simulink model "DC_motor_PID"  (R2024a)
settings: Solver=VariableStepAuto  StartTime=0.0  StopTime=10.0  RelTol=1e-3
libraries: simulink_extras x4, nesl_utility x4, fl_lib x2
settings Model: Creator=fuad  LastModifiedBy=fuad

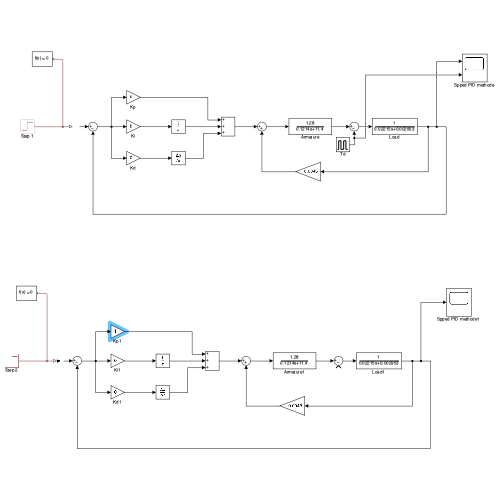
[thumbnail: Simulink's stored preview of the top-level diagram]
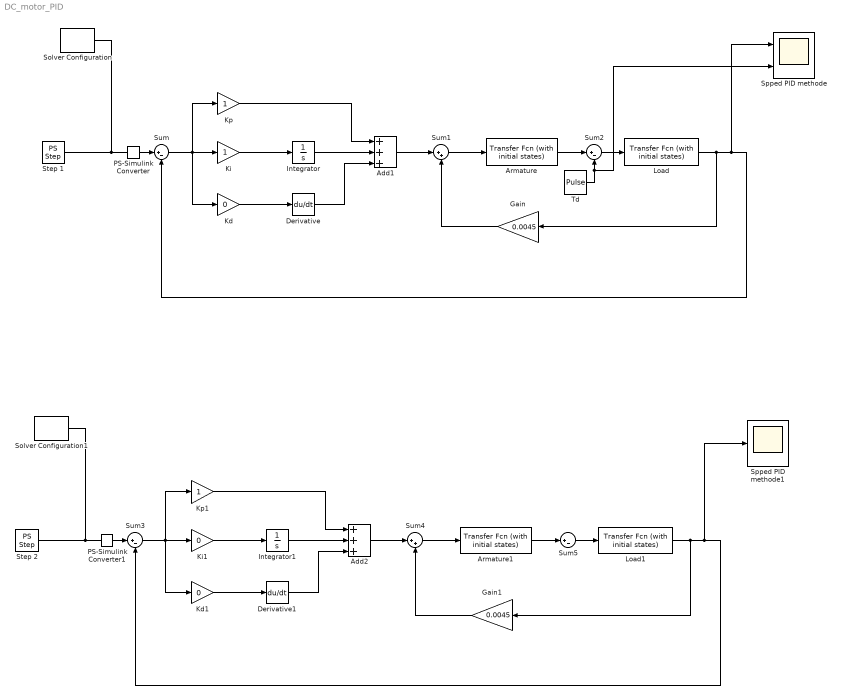
== system DC_motor_PID ==
  Add1 : Sum  Inputs=+++
  Add2 : Sum  Inputs=+++
  Armature : simulink_extras/Additional Linear/Transfer Fcn (with initial states)  N=[1.28]  D="[0.1214  11.4]"  X0=.0
  Armature1 : simulink_extras/Additional Linear/Transfer Fcn (with initial states)  N=[1.28]  D="[0.1214  11.4]"  X0=.0
  Derivative : Derivative
  Derivative1 : Derivative
  Gain : Gain  Gain=0.0045
  Gain1 : Gain  Gain=0.0045
  Integrator : Integrator
  Integrator1 : Integrator
  Kd : Gain  Gain=0
  Kd1 : Gain  Gain=0
  Ki : Gain
  Ki1 : Gain  Gain=0
  Kp : Gain
  Kp1 : Gain
  Load : simulink_extras/Additional Linear/Transfer Fcn (with initial states)  N=[1]  D="[0.02215  0.002953]"  X0=.0
  Load1 : simulink_extras/Additional Linear/Transfer Fcn (with initial states)  N=[1]  D="[0.02215  0.002953]"  X0=.0
  PS-Simulink Converter : nesl_utility/PS-Simulink Converter  PhysicalDomain=network_engine_domain  SubClassName=ps_output  LeftPortType=input  RightPortType=output  PseudoPeriodic=off  Frequencies=[]  VectorFormat=inherit  Unit=inherit  AffineConversion=off
  PS-Simulink Converter1 : nesl_utility/PS-Simulink Converter  PhysicalDomain=network_engine_domain  SubClassName=ps_output  LeftPortType=input  RightPortType=output  PseudoPeriodic=off  Frequencies=[]  VectorFormat=inherit  Unit=inherit  AffineConversion=off
  Solver Configuration : nesl_utility/Solver Configuration  PhysicalDomain=network_engine_domain  SubClassName=solver  LeftPortType=input  RightPortType=generic  Tones=[]  Harmonics=[]  SimulateNoise=off  Profile=off  UseLocalSampling=off  EnableSwitchedLinearOptims=on  FrequencyDomain=off  UseCCode=off  RelTol=0.001  AbsTol=0.001  MinStep=1e-09  ToWorkspace=off  RevertToSquareIcSolve=off  NumHomotopyIterations=100  PhasorMode=off  PhasorModeNumHarmonics=1  ConsistencySolver=NEWTON_XTOL_AFTER_FTOL  IndexReductionMethod=DerivativeReplacement  DoDC=off  ResidualTolerance=1e-09  ConsistencyTolSource=GLOBAL  ConsistencyAbsTol=0.001  ConsistencyRelTol=0.001  ConsistencyTolFactor=0.001  UseLocalSolver=off  LocalSolverChoice=NE_BACKWARD_EULER_ADVANCER  ResolveIndetEquations=on  FunctionEvalNumThread=1  LocalSolverSampleTime=0.001  DoFixedCost=off  MaxNonlinIter=3  MaxModeIter=2  ComputeImpulses=off  ImpulseIterations=2  LinearAlgebra=auto  LinearAlgebraNumThread=0  EquationFormulation=NE_TIME_EF  DelaysMemoryBudget=1024  AutomaticFiltering=on  FilteringTimeConstant=0.001  PartitionStorageMethod=AS_NEEDED  PartitionMemoryBudget=1024  PartitionMethod=ROBUST  MultibodyUseLocalSolver=off  MultibodyLocalSolverChoice=ODE1  MultibodyLocalSolverSampleTime=0.001
  Solver Configuration1 : nesl_utility/Solver Configuration  PhysicalDomain=network_engine_domain  SubClassName=solver  LeftPortType=input  RightPortType=generic  Tones=[]  Harmonics=[]  SimulateNoise=off  Profile=off  UseLocalSampling=off  EnableSwitchedLinearOptims=on  FrequencyDomain=off  UseCCode=off  RelTol=0.001  AbsTol=0.001  MinStep=1e-09  ToWorkspace=off  RevertToSquareIcSolve=off  NumHomotopyIterations=100  PhasorMode=off  PhasorModeNumHarmonics=1  ConsistencySolver=NEWTON_XTOL_AFTER_FTOL  IndexReductionMethod=DerivativeReplacement  DoDC=off  ResidualTolerance=1e-09  ConsistencyTolSource=GLOBAL  ConsistencyAbsTol=0.001  ConsistencyRelTol=0.001  ConsistencyTolFactor=0.001  UseLocalSolver=off  LocalSolverChoice=NE_BACKWARD_EULER_ADVANCER  ResolveIndetEquations=on  FunctionEvalNumThread=1  LocalSolverSampleTime=0.001  DoFixedCost=off  MaxNonlinIter=3  MaxModeIter=2  ComputeImpulses=off  ImpulseIterations=2  LinearAlgebra=auto  LinearAlgebraNumThread=0  EquationFormulation=NE_TIME_EF  DelaysMemoryBudget=1024  AutomaticFiltering=on  FilteringTimeConstant=0.001  PartitionStorageMethod=AS_NEEDED  PartitionMemoryBudget=1024  PartitionMethod=ROBUST  MultibodyUseLocalSolver=off  MultibodyLocalSolverChoice=ODE1  MultibodyLocalSolverSampleTime=0.001
  Spped PID methode : Scope  NumInputPorts=2
  Spped PID methode1 : Scope
  Step 1 : fl_lib/Physical Signals/Sources/PS Step  step_time=0 s  initial_value=0  final_value=1
  Step 2 : fl_lib/Physical Signals/Sources/PS Step  step_time=0 s  initial_value=0  final_value=1
  Sum{,2..3,5} (4 alike) : Sum  Inputs=|+-
  Sum1 : Sum  Inputs=|++
  Sum4 : Sum  Inputs=|++
  Td : DiscretePulseGenerator  PulseType=Time based  Amplitude=0.03  Period=10  PulseWidth=10  PhaseDelay=1
  wires:
  PS-Simulink Converter/1 -> Sum/1
  Sum/1 -> Kd/1, Ki/1, Kp/1
  Ki/1 -> Integrator/1
  Kd/1 -> Derivative/1
  Kp/1 -> Add1/1
  Integrator/1 -> Add1/2
  Derivative/1 -> Add1/3
  Add1/1 -> Sum1/1
  Sum1/1 -> Armature/1
  Load/1 -> Gain/1, Spped PID methode/1, Sum/2
  Armature/1 -> Sum2/1
  Sum2/1 -> Load/1
  Gain/1 -> Sum1/2
  Td/1 -> Spped PID methode/2, Sum2/2
  Gain1/1 -> Sum4/2
  Derivative1/1 -> Add2/3
  Armature1/1 -> Sum5/1
  Sum5/1 -> Load1/1
  Kd1/1 -> Derivative1/1
  Integrator1/1 -> Add2/2
  PS-Simulink Converter1/1 -> Sum3/1
  Ki1/1 -> Integrator1/1
  Sum4/1 -> Armature1/1
  Kp1/1 -> Add2/1
  Load1/1 -> Gain1/1, Spped PID methode1/1, Sum3/2
  Add2/1 -> Sum4/1
  Sum3/1 -> Kd1/1, Ki1/1, Kp1/1
  connections:
  PS-Simulink Converter/LConn1 -- Step 1/RConn1 -- Solver Configuration/RConn1
  PS-Simulink Converter1/LConn1 -- Step 2/RConn1 -- Solver Configuration1/RConn1
